simulink model "aaa"  (R2016b)
settings: Solver=ode4  StartTime=0.0  StopTime=inf  FixedStep=0.002  RelTol=1e-3  EnableMultiTasking=on
libraries: slrtlib x3
(part 2 of 5)

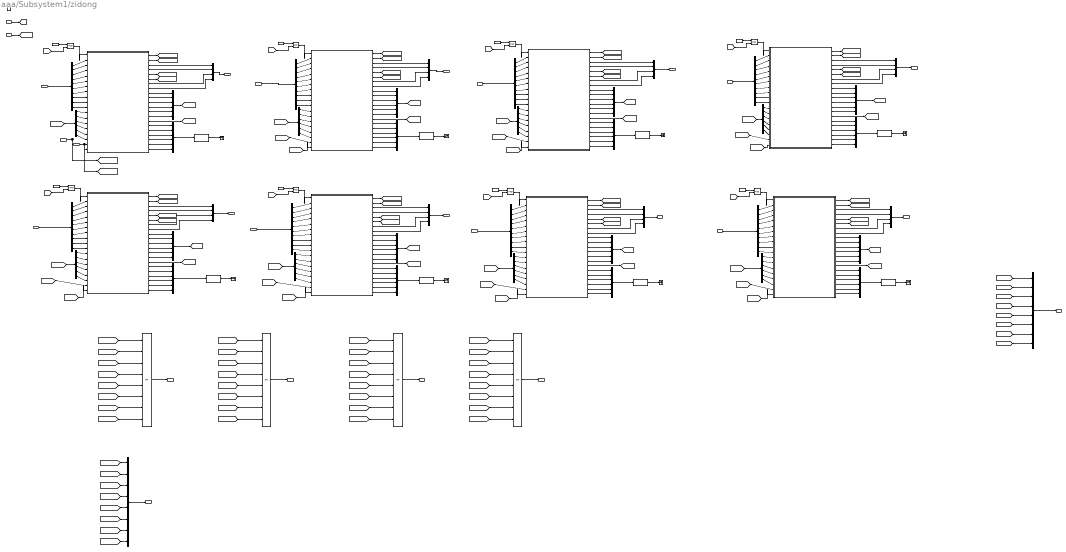
== system aaa/Subsystem1/zidong ==
  start : Inport
  In1 : Inport  Port=2
  In2 : Inport  Port=3
  In3 : Inport  Port=4
  In4 : Inport  Port=5
  In5 : Inport  Port=6
  In6 : Inport  Port=7
  In7 : Inport  Port=8
  In8 : Inport  Port=9
  "jiangeshijian " : Inport  Port=10
  shedingcishu : Inport  Port=11
  jieshu : Inport  Port=12
  Enable : EnablePort
  1# : Stateflow chart  TreatAsAtomicUnit=on
  1#1 : Stateflow chart  TreatAsAtomicUnit=on
  1#2 : Stateflow chart  TreatAsAtomicUnit=on
  1#3 : Stateflow chart  TreatAsAtomicUnit=on
  1#4 : Stateflow chart  TreatAsAtomicUnit=on
  1#5 : Stateflow chart  TreatAsAtomicUnit=on
  1#6 : Stateflow chart  TreatAsAtomicUnit=on
  1#7 : Stateflow chart  TreatAsAtomicUnit=on
  Data Type Conversion{1..8} (8 alike) : DataTypeConversion
  Demux{1..2,4,6,8,12,14,16} (8 alike) : Demux  Outputs=6
  Demux{3,5,7,9..11,13,15} (8 alike) : Demux  Outputs=10
  Logical Operator{,1..3} (4 alike) : Logic  Operator=OR  Inputs=8  AllPortsSameDT=off  OutDataTypeStr=boolean
  Logical Operator{4..11} (8 alike) : Logic  AllPortsSameDT=off  OutDataTypeStr=boolean
  Mux{,1..7} (8 alike) : Mux
  Mux{8..15,18..25} (16 alike) : Mux  Inputs=6
  Mux16 : Mux  Inputs=8
  Mux17 : Mux  Inputs=8
  Terminator{,1..7} (8 alike) : Terminator
  kaishi{1..8} (8 alike) : Constant  Value=0
      settings: OpenFcn=|
      | if get_param(gcb,'value')=='1',
      | set_param(gcb,'value','0');
      | else
      | set_param(gcb,'value','1');end
  songkaihuanxiang : Outport
  kaigaihuanxiang : Outport  Port=2
  yajinhuanxiang : Outport  Port=3
  guangaihuanxiang : Outport  Port=4
  Out1 : Outport  Port=5
  Out2 : Outport  Port=6
  Out3 : Outport  Port=7
  Out4 : Outport  Port=8
  Out5 : Outport  Port=9
  Out6 : Outport  Port=10
  Out7 : Outport  Port=11
  Out8 : Outport  Port=12
  "zidongshijian " : Outport  Port=13
  yikaicishu : Outport  Port=14
  wires:
  "jiangeshijian "/1 -> [jiangeshijian]
  Demux1/1 -> 1#/12(t1)
  Demux1/2 -> 1#/13(t3)
  Demux1/3 -> 1#/14(t5)
  Demux1/4 -> 1#/15(t7)
  Demux1/5 -> 1#/16(t9)
  [jiangeshijian] -> Demux1/1
  Demux9/1 -> 1#/2(kgdw1)
  Demux9/2 -> 1#/3(kgdw2)
  Demux9/3 -> 1#/4(ggdw1)
  Demux9/4 -> 1#/5(ggdw2)
  Demux9/5 -> 1#/6(kghc)
  Demux9/6 -> 1#/7(gghc)
  Demux9/7 -> 1#/8(sddw)
  Demux9/8 -> 1#/9(yjdw)
  Demux9/9 -> 1#/10(skdw)
  Demux9/10 -> 1#/11(jsdw)
  In1/1 -> Demux9/1  "kaigaidaowei1 kaigaidaowei2 guangaidaowei1 guangaidaowei2 kaigaihuanchong guangaihuanchong suodingdaowei jiesuodaowei yajindaowei songkaidaowei"
  start/1 -> [start]
  [start] -> Logical Operator4/2
  Demux2/1 -> 1#1/12(t1)
  Demux2/2 -> 1#1/13(t3)
  Demux2/3 -> 1#1/14(t5)
  Demux2/4 -> 1#1/15(t7)
  Demux2/5 -> 1#1/16(t9)
  [jiangeshijian] -> Demux2/1
  Demux3/1 -> 1#1/2(kgdw1)
  Demux3/2 -> 1#1/3(kgdw2)
  Demux3/3 -> 1#1/4(ggdw1)
  Demux3/4 -> 1#1/5(ggdw2)
  Demux3/5 -> 1#1/6(kghc)
  Demux3/6 -> 1#1/7(gghc)
  Demux3/7 -> 1#1/8(sddw)
  Demux3/8 -> 1#1/9(yjdw)
  Demux3/9 -> 1#1/10(skdw)
  Demux3/10 -> 1#1/11(jsdw)
  In2/1 -> Demux3/1  "kaigaidaowei1 kaigaidaowei2 guangaidaowei1 guangaidaowei2 kaigaihuanchong guangaihuanchong suodingdaowei jiesuodaowei yajindaowei songkaidaowei"
  [jiangeshijian] -> Demux4/1
  In3/1 -> Demux5/1  "kaigaidaowei1 kaigaidaowei2 guangaidaowei1 guangaidaowei2 kaigaihuanchong guangaihuanchong suodingdaowei jiesuodaowei yajindaowei songkaidaowei"
  [jiangeshijian] -> Demux6/1
  In4/1 -> Demux7/1  "kaigaidaowei1 kaigaidaowei2 guangaidaowei1 guangaidaowei2 kaigaihuanchong guangaihuanchong suodingdaowei jiesuodaowei yajindaowei songkaidaowei"
  [jiangeshijian] -> Demux8/1
  In5/1 -> Demux10/1  "kaigaidaowei1 kaigaidaowei2 guangaidaowei1 guangaidaowei2 kaigaihuanchong guangaihuanchong suodingdaowei jiesuodaowei yajindaowei songkaidaowei"
  [jiangeshijian] -> Demux12/1
  In6/1 -> Demux11/1  "kaigaidaowei1 kaigaidaowei2 guangaidaowei1 guangaidaowei2 kaigaihuanchong guangaihuanchong suodingdaowei jiesuodaowei yajindaowei songkaidaowei"
  [jiangeshijian] -> Demux14/1
  In7/1 -> Demux13/1  "kaigaidaowei1 kaigaidaowei2 guangaidaowei1 guangaidaowei2 kaigaihuanchong guangaihuanchong suodingdaowei jiesuodaowei yajindaowei songkaidaowei"
  [jiangeshijian] -> Demux16/1
  In8/1 -> Demux15/1  "kaigaidaowei1 kaigaidaowei2 guangaidaowei1 guangaidaowei2 kaigaihuanchong guangaihuanchong suodingdaowei jiesuodaowei yajindaowei songkaidaowei"
  Demux15/1 -> 1#7/2(kgdw1)
  Demux15/2 -> 1#7/3(kgdw2)
  Demux15/3 -> 1#7/4(ggdw1)
  Demux15/4 -> 1#7/5(ggdw2)
  Demux15/5 -> 1#7/6(kghc)
  Demux15/6 -> 1#7/7(gghc)
  Demux15/7 -> 1#7/8(sddw)
  Demux15/8 -> 1#7/9(yjdw)
  Demux15/9 -> 1#7/10(skdw)
  Demux15/10 -> 1#7/11(jsdw)
  Demux16/1 -> 1#7/12(t1)
  Demux16/2 -> 1#7/13(t3)
  Demux16/3 -> 1#7/14(t5)
  Demux16/4 -> 1#7/15(t7)
  Demux16/5 -> 1#7/16(t9)
  Demux13/1 -> 1#6/2(kgdw1)
  Demux13/2 -> 1#6/3(kgdw2)
  Demux13/3 -> 1#6/4(ggdw1)
  Demux13/4 -> 1#6/5(ggdw2)
  Demux13/5 -> 1#6/6(kghc)
  Demux13/6 -> 1#6/7(gghc)
  Demux13/7 -> 1#6/8(sddw)
  Demux13/8 -> 1#6/9(yjdw)
  Demux13/9 -> 1#6/10(skdw)
  Demux13/10 -> 1#6/11(jsdw)
  Demux14/1 -> 1#6/12(t1)
  Demux14/2 -> 1#6/13(t3)
  Demux14/3 -> 1#6/14(t5)
  Demux14/4 -> 1#6/15(t7)
  Demux14/5 -> 1#6/16(t9)
  Demux11/1 -> 1#5/2(kgdw1)
  Demux11/2 -> 1#5/3(kgdw2)
  Demux11/3 -> 1#5/4(ggdw1)
  Demux11/4 -> 1#5/5(ggdw2)
  Demux11/5 -> 1#5/6(kghc)
  Demux11/6 -> 1#5/7(gghc)
  Demux11/7 -> 1#5/8(sddw)
  Demux11/8 -> 1#5/9(yjdw)
  Demux11/9 -> 1#5/10(skdw)
  Demux11/10 -> 1#5/11(jsdw)
  Demux12/5 -> 1#5/16(t9)
  Demux12/4 -> 1#5/15(t7)
  Demux12/3 -> 1#5/14(t5)
  Demux12/1 -> 1#5/12(t1)
  Demux12/2 -> 1#5/13(t3)
  Demux8/1 -> 1#4/12(t1)
  Demux8/2 -> 1#4/13(t3)
  Demux8/3 -> 1#4/14(t5)
  Demux8/4 -> 1#4/15(t7)
  Demux8/5 -> 1#4/16(t9)
  Demux10/1 -> 1#4/2(kgdw1)
  Demux10/2 -> 1#4/3(kgdw2)
  Demux10/3 -> 1#4/4(ggdw1)
  Demux10/4 -> 1#4/5(ggdw2)
  Demux10/5 -> 1#4/6(kghc)
  Demux10/6 -> 1#4/7(gghc)
  Demux10/7 -> 1#4/8(sddw)
  Demux10/8 -> 1#4/9(yjdw)
  Demux10/9 -> 1#4/10(skdw)
  Demux10/10 -> 1#4/11(jsdw)
  Demux5/1 -> 1#2/2(kgdw1)
  Demux5/2 -> 1#2/3(kgdw2)
  Demux5/3 -> 1#2/4(ggdw1)
  Demux5/4 -> 1#2/5(ggdw2)
  Demux5/5 -> 1#2/6(kghc)
  Demux5/6 -> 1#2/7(gghc)
  Demux5/7 -> 1#2/8(sddw)
  Demux5/8 -> 1#2/9(yjdw)
  Demux5/9 -> 1#2/10(skdw)
  Demux5/10 -> 1#2/11(jsdw)
  Demux4/1 -> 1#2/12(t1)
  Demux4/2 -> 1#2/13(t3)
  Demux4/3 -> 1#2/14(t5)
  Demux4/4 -> 1#2/15(t7)
  Demux4/5 -> 1#2/16(t9)
  Demux7/1 -> 1#3/2(kgdw1)
  Demux7/2 -> 1#3/3(kgdw2)
  Demux7/3 -> 1#3/4(ggdw1)
  Demux7/4 -> 1#3/5(ggdw2)
  Demux7/5 -> 1#3/6(kghc)
  Demux7/6 -> 1#3/7(gghc)
  Demux7/7 -> 1#3/8(sddw)
  Demux7/8 -> 1#3/9(yjdw)
  Demux7/9 -> 1#3/10(skdw)
  Demux7/10 -> 1#3/11(jsdw)
  Demux6/1 -> 1#3/12(t1)
  Demux6/2 -> 1#3/13(t3)
  Demux6/3 -> 1#3/14(t5)
  Demux6/4 -> 1#3/15(t7)
  Demux6/5 -> 1#3/16(t9)
  1#/1(skhx) -> [songkaihuanxiang1]
  1#/2(kghx) -> [kaigaihuanxiang1]
  1#/5(yjhx) -> [yajinhuanxiang1]
  1#/6(gghx) -> [guangaihuanxiang1]
  1#1/1(skhx) -> [songkaihuanxiang2]
  1#1/2(kghx) -> [kaigaihuanxiang2]
  1#1/5(yjhx) -> [yajinhuanxiang2]
  1#1/6(gghx) -> [guangaihuanxiang2]
  1#2/1(skhx) -> [songkaihuanxiang3]
  1#2/2(kghx) -> [kaigaihuanxiang3]
  1#2/5(yjhx) -> [yajinhuanxiang3]
  1#2/6(gghx) -> [guangaihuanxiang3]
  1#4/2(kghx) -> [kaigaihuanxiang5]
  1#4/1(skhx) -> [songkaihuanxiang5]
  1#5/1(skhx) -> [songkaihuanxiang6]
  1#5/2(kghx) -> [kaigaihuanxiang6]
  1#7/1(skhx) -> [songkaihuanxiang8]
  1#7/2(kghx) -> [kaigaihuanxiang8]
  1#6/1(skhx) -> [songkaihuanxiang7]
  1#6/2(kghx) -> [kaigaihuanxiang7]
  1#6/5(yjhx) -> [yajinhuanxiang7]
  1#6/6(gghx) -> [guangaihuanxiang7]
  1#3/1(skhx) -> [songkaihuanxiang4]
  1#3/2(kghx) -> [kaigaihuanxiang4]
  [songkaihuanxiang1] -> Logical Operator/1
  [songkaihuanxiang2] -> Logical Operator/2
  [songkaihuanxiang3] -> Logical Operator/3
  [songkaihuanxiang4] -> Logical Operator/4
  [songkaihuanxiang5] -> Logical Operator/5
  [songkaihuanxiang8] -> Logical Operator/8
  [songkaihuanxiang7] -> Logical Operator/7
  [songkaihuanxiang6] -> Logical Operator/6
  Logical Operator/1 -> songkaihuanxiang/1
  [kaigaihuanxiang1] -> Logical Operator1/1
  [kaigaihuanxiang2] -> Logical Operator1/2
  [kaigaihuanxiang3] -> Logical Operator1/3
  [kaigaihuanxiang4] -> Logical Operator1/4
  [kaigaihuanxiang5] -> Logical Operator1/5
  [kaigaihuanxiang8] -> Logical Operator1/8
  [kaigaihuanxiang7] -> Logical Operator1/7
  [kaigaihuanxiang6] -> Logical Operator1/6
  Logical Operator1/1 -> kaigaihuanxiang/1
  [yajinhuanxiang1] -> Logical Operator2/1
  [yajinhuanxiang2] -> Logical Operator2/2
  [yajinhuanxiang3] -> Logical Operator2/3
  [yajinhuanxiang4] -> Logical Operator2/4
  [yajinhuanxiang5] -> Logical Operator2/5
  [yajinhuanxiang8] -> Logical Operator2/8
  [yajinhuanxiang7] -> Logical Operator2/7
  [yajinhuanxiang6] -> Logical Operator2/6
  Logical Operator2/1 -> yajinhuanxiang/1
  [guangaihuanxiang1] -> Logical Operator3/1
  [guangaihuanxiang2] -> Logical Operator3/2
  [guangaihuanxiang3] -> Logical Operator3/3
  [guangaihuanxiang4] -> Logical Operator3/4
  [guangaihuanxiang5] -> Logical Operator3/5
  [guangaihuanxiang8] -> Logical Operator3/8
  [guangaihuanxiang7] -> Logical Operator3/7
  [guangaihuanxiang6] -> Logical Operator3/6
  Logical Operator3/1 -> guangaihuanxiang/1
  1#/3(kgzhiling1) -> Mux/1
  1#/4(kgzhiling2) -> Mux/2
  1#/7(ggzhiling1) -> Mux/3
  1#/8(ggzhiling2) -> Mux/4
  1#1/7(ggzhiling1) -> Mux1/3
  Mux/1 -> Out1/1
  Mux1/1 -> Out2/1
  Mux2/1 -> Out3/1
  Mux4/1 -> Out5/1
  1#/9(skt) -> Mux8/1
  1#/10(kgt) -> Mux8/2
  1#/11(sdt) -> Mux8/3
  1#/12(jst) -> Mux8/4
  1#/13(ggt) -> Mux8/5
  1#/14(yjt) -> Mux8/6
  Mux8/1 -> [shijian1]
  Mux11/1 -> [shijian4]
  Mux21/1 -> [shijian5]
  [shijian1] -> Mux16/1
  [shijian2] -> Mux16/2
  [shijian3] -> Mux16/3
  [shijian4] -> Mux16/4
  [shijian5] -> Mux16/5
  [shijian6] -> Mux16/6
  [shijian7] -> Mux16/7
  Mux16/1 -> "zidongshijian "/1
  [shedingcishu] -> 1#5/18(shedingcishu)
  [shedingcishu] -> 1#6/18(shedingcishu)
  [shedingcishu] -> 1#7/18(shedingcishu)
  shedingcishu/1 -> 1#/18(shedingcishu), [shedingcishu]
  [shedingcishu] -> 1#4/18(shedingcishu)
  [shedingcishu] -> 1#1/18(shedingcishu)
  [shedingcishu] -> 1#2/18(shedingcishu)
  [shedingcishu] -> 1#3/18(shedingcishu)
  1#/15(yikaicishu) -> [yikaicishu1]
  1#1/15(yikaicishu) -> [yikaicishu2]
  1#2/15(yikaicishu) -> [yikaicishu3]
  [yikaicishu1] -> Mux17/1
  [yikaicishu4] -> Mux17/4
  [yikaicishu8] -> Mux17/8
  [yikaicishu7] -> Mux17/7
  [yikaicishu6] -> Mux17/6
  [yikaicishu5] -> Mux17/5
  [yikaicishu2] -> Mux17/2
  [yikaicishu3] -> Mux17/3
  Mux17/1 -> yikaicishu/1
  jieshu/1 -> 1#/19(jieshu), [jieshu]
  [jieshu] -> 1#1/19(jieshu)
  [jieshu] -> 1#2/19(jieshu)
  [jieshu] -> 1#3/19(jieshu)
  [jieshu] -> 1#7/19(jieshu)
  [jieshu] -> 1#4/19(jieshu)
  [jieshu] -> 1#5/19(jieshu)
  [jieshu] -> 1#6/19(jieshu)
  kaishi1/1 -> Logical Operator4/1
  Logical Operator4/1 -> 1#/1(start)
  [start] -> Logical Operator5/2
  kaishi2/1 -> Logical Operator5/1
  Logical Operator5/1 -> 1#1/1(start)
  [start] -> Logical Operator6/2
  kaishi3/1 -> Logical Operator6/1
  Logical Operator6/1 -> 1#2/1(start)
  [start] -> Logical Operator7/2
  kaishi4/1 -> Logical Operator7/1
  Logical Operator7/1 -> 1#3/1(start)
  [start] -> Logical Operator8/2
  kaishi5/1 -> Logical Operator8/1
  Logical Operator8/1 -> 1#4/1(start)
  [start] -> Logical Operator9/2
  kaishi6/1 -> Logical Operator9/1
  Logical Operator9/1 -> 1#5/1(start)
  [start] -> Logical Operator10/2
  kaishi7/1 -> Logical Operator10/1
  Logical Operator10/1 -> 1#6/1(start)
  [start] -> Logical Operator11/2
  kaishi8/1 -> Logical Operator11/1
  Logical Operator11/1 -> 1#7/1(start)
  Demux1/6 -> 1#/17(t11)
  Demux2/6 -> 1#1/17(t11)
  Demux4/6 -> 1#2/17(t11)
  Demux6/6 -> 1#3/17(t11)
  Demux8/6 -> 1#4/17(t11)
  Demux12/6 -> 1#5/17(t11)
  Demux14/6 -> 1#6/17(t11)
  Demux16/6 -> 1#7/17(t11)
  1#/16(skyichang) -> Mux18/1
  1#/17(kgyichang) -> Mux18/2
  1#/18(sdyichang) -> Mux18/3
  1#/19(jsyichang) -> Mux18/4
  1#/20(ggyichang) -> Mux18/5
  1#/21(yjyichang) -> Mux18/6
  Mux18/1 -> Data Type Conversion1/1
  Data Type Conversion1/1 -> Terminator/1
  1#1/3(kgzhiling1) -> Mux1/1
  1#1/4(kgzhiling2) -> Mux1/2
  1#1/8(ggzhiling2) -> Mux1/4
  1#1/9(skt) -> Mux9/1
  1#1/10(kgt) -> Mux9/2
  1#1/11(sdt) -> Mux9/3
  1#1/12(jst) -> Mux9/4
  1#1/13(ggt) -> Mux9/5
  1#1/14(yjt) -> Mux9/6
  Mux9/1 -> [shijian2]
  1#1/16(skyichang) -> Mux19/1
  1#1/17(kgyichang) -> Mux19/2
  1#1/18(sdyichang) -> Mux19/3
  1#1/19(jsyichang) -> Mux19/4
  1#1/20(ggyichang) -> Mux19/5
  1#1/21(yjyichang) -> Mux19/6
  Mux19/1 -> Data Type Conversion2/1
  Data Type Conversion2/1 -> Terminator1/1
  1#2/3(kgzhiling1) -> Mux2/1
  1#2/4(kgzhiling2) -> Mux2/2
  1#2/7(ggzhiling1) -> Mux2/3
  1#2/8(ggzhiling2) -> Mux2/4
  1#2/9(skt) -> Mux10/1
  1#2/10(kgt) -> Mux10/2
  1#2/11(sdt) -> Mux10/3
  1#2/12(jst) -> Mux10/4
  1#2/13(ggt) -> Mux10/5
  1#2/14(yjt) -> Mux10/6
  Mux10/1 -> [shijian3]
  1#2/16(skyichang) -> Mux20/1
  1#2/17(kgyichang) -> Mux20/2
  1#2/18(sdyichang) -> Mux20/3
  1#2/19(jsyichang) -> Mux20/4
  1#2/20(ggyichang) -> Mux20/5
  1#2/21(yjyichang) -> Mux20/6
  Mux20/1 -> Data Type Conversion3/1
  Data Type Conversion3/1 -> Terminator2/1
  1#3/5(yjhx) -> [yajinhuanxiang4]
  1#3/6(gghx) -> [guangaihuanxiang4]
  Mux3/1 -> Out4/1
  1#3/3(kgzhiling1) -> Mux3/1
  1#3/4(kgzhiling2) -> Mux3/2
  1#3/7(ggzhiling1) -> Mux3/3
  1#3/8(ggzhiling2) -> Mux3/4
  1#4/6(gghx) -> [guangaihuanxiang5]
  1#4/5(yjhx) -> [yajinhuanxiang5]
  1#4/3(kgzhiling1) -> Mux4/1
  1#4/4(kgzhiling2) -> Mux4/2
  1#4/7(ggzhiling1) -> Mux4/3
  1#4/8(ggzhiling2) -> Mux4/4
  1#4/9(skt) -> Mux21/1
  1#4/10(kgt) -> Mux21/2
  1#4/11(sdt) -> Mux21/3
  1#4/12(jst) -> Mux21/4
  1#4/13(ggt) -> Mux21/5
  1#4/14(yjt) -> Mux21/6
  1#4/15(yikaicishu) -> [yikaicishu5]
  1#4/17(kgyichang) -> Mux14/2
  1#4/18(sdyichang) -> Mux14/3
  1#4/19(jsyichang) -> Mux14/4
  1#4/20(ggyichang) -> Mux14/5
  1#4/21(yjyichang) -> Mux14/6
  1#4/16(skyichang) -> Mux14/1
  Mux14/1 -> Data Type Conversion4/1
  Data Type Conversion4/1 -> Terminator3/1
  1#5/15(yikaicishu) -> [yikaicishu6]
  1#5/5(yjhx) -> [yajinhuanxiang6]
  1#5/6(gghx) -> [guangaihuanxiang6]
  1#5/7(ggzhiling1) -> Mux5/3
  Mux5/1 -> Out6/1
  1#5/3(kgzhiling1) -> Mux5/1
  1#5/4(kgzhiling2) -> Mux5/2
  1#5/8(ggzhiling2) -> Mux5/4
  1#5/9(skt) -> Mux15/1
  1#5/10(kgt) -> Mux15/2
  1#5/11(sdt) -> Mux15/3
  1#5/12(jst) -> Mux15/4
  1#5/13(ggt) -> Mux15/5
  1#5/14(yjt) -> Mux15/6
  Mux15/1 -> [shijian6]
  1#5/16(skyichang) -> Mux22/1
  1#5/17(kgyichang) -> Mux22/2
  1#5/18(sdyichang) -> Mux22/3
  1#5/19(jsyichang) -> Mux22/4
  1#5/20(ggyichang) -> Mux22/5
  1#5/21(yjyichang) -> Mux22/6
  Mux22/1 -> Data Type Conversion5/1
  Data Type Conversion5/1 -> Terminator4/1
  1#6/7(ggzhiling1) -> Mux6/3
  Mux6/1 -> Out7/1
  1#6/3(kgzhiling1) -> Mux6/1
  1#6/4(kgzhiling2) -> Mux6/2
  1#6/8(ggzhiling2) -> Mux6/4
  1#6/9(skt) -> Mux12/1
  1#6/10(kgt) -> Mux12/2
  1#6/11(sdt) -> Mux12/3
  1#6/12(jst) -> Mux12/4
  1#6/13(ggt) -> Mux12/5
  1#6/14(yjt) -> Mux12/6
  Mux12/1 -> [shijian7]
  1#6/15(yikaicishu) -> [yikaicishu7]
  1#6/16(skyichang) -> Mux23/1
  1#6/17(kgyichang) -> Mux23/2
  1#6/18(sdyichang) -> Mux23/3
  1#6/19(jsyichang) -> Mux23/4
  1#6/20(ggyichang) -> Mux23/5
  1#6/21(yjyichang) -> Mux23/6
  Mux23/1 -> Data Type Conversion6/1
  Data Type Conversion6/1 -> Terminator5/1
  1#7/5(yjhx) -> [yajinhuanxiang8]
  1#7/6(gghx) -> [guangaihuanxiang8]
  1#7/7(ggzhiling1) -> Mux7/3
  Mux7/1 -> Out8/1
  1#7/3(kgzhiling1) -> Mux7/1
  1#7/4(kgzhiling2) -> Mux7/2
  1#7/8(ggzhiling2) -> Mux7/4
  1#7/9(skt) -> Mux13/1
  1#7/10(kgt) -> Mux13/2
  1#7/11(sdt) -> Mux13/3
  1#7/12(jst) -> Mux13/4
  1#7/13(ggt) -> Mux13/5
  1#7/14(yjt) -> Mux13/6
  Mux13/1 -> [shijian8]
  1#7/15(yikaicishu) -> [yikaicishu8]
  1#7/16(skyichang) -> Mux24/1
  1#7/17(kgyichang) -> Mux24/2
  1#7/18(sdyichang) -> Mux24/3
  1#7/19(jsyichang) -> Mux24/4
  1#7/20(ggyichang) -> Mux24/5
  1#7/21(yjyichang) -> Mux24/6
  Mux24/1 -> Data Type Conversion7/1
  Data Type Conversion7/1 -> Terminator6/1
  [shijian8] -> Mux16/8
  1#3/15(yikaicishu) -> [yikaicishu4]
  1#3/9(skt) -> Mux11/1
  1#3/10(kgt) -> Mux11/2
  1#3/11(sdt) -> Mux11/3
  1#3/12(jst) -> Mux11/4
  1#3/13(ggt) -> Mux11/5
  1#3/14(yjt) -> Mux11/6
  1#3/16(skyichang) -> Mux25/1
  1#3/17(kgyichang) -> Mux25/2
  1#3/18(sdyichang) -> Mux25/3
  1#3/19(jsyichang) -> Mux25/4
  1#3/20(ggyichang) -> Mux25/5
  1#3/21(yjyichang) -> Mux25/6
  Mux25/1 -> Data Type Conversion8/1
  Data Type Conversion8/1 -> Terminator7/1

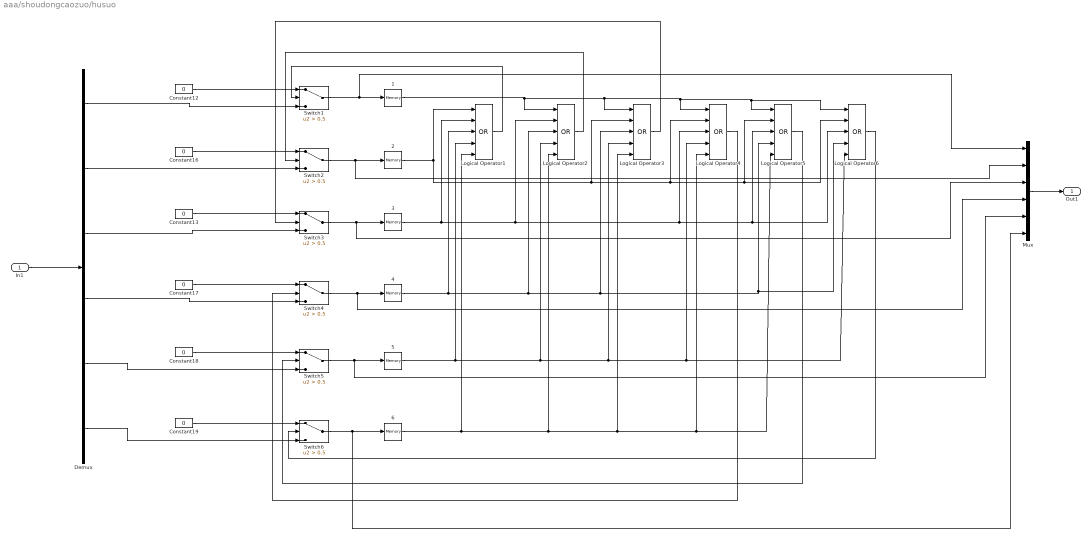
== system aaa/shoudongcaozuo/husuo ==
  In1 : Inport
  {1..6} (6 alike) : Memory
  Constant{12..13,16..19} (6 alike) : Constant  Value=0
  Demux : Demux  Outputs=6
  Logical Operator{1..6} (6 alike) : Logic  Operator=OR  Inputs=5  AllPortsSameDT=off  OutDataTypeStr=boolean
  Mux : Mux  Inputs=6
  Switch{1..6} (6 alike) : Switch  Criteria=u2 > Threshold  Threshold=0.5
  Out1 : Outport
  wires:
  In1/1 -> Demux/1
  Mux/1 -> Out1/1
  Constant16/1 -> Switch2/1
  Constant12/1 -> Switch1/1
  Constant17/1 -> Switch4/1
  Constant13/1 -> Switch3/1
  Constant19/1 -> Switch6/1
  Constant18/1 -> Switch5/1
  Switch1/1 -> Mux/1, 1/1
  Switch2/1 -> Mux/2, 2/1
  Switch3/1 -> Mux/3, 3/1
  Switch4/1 -> Mux/4, 4/1
  Switch5/1 -> Mux/5, 5/1
  Switch6/1 -> Mux/6, 6/1
  2/1 -> Logical Operator6/2, Logical Operator5/2, Logical Operator4/2, Logical Operator3/2, Logical Operator1/1
  3/1 -> Logical Operator6/3, Logical Operator5/3, Logical Operator4/3, Logical Operator2/2, Logical Operator1/2
  4/1 -> Logical Operator6/4, Logical Operator5/4, Logical Operator3/3, Logical Operator2/3, Logical Operator1/3
  5/1 -> Logical Operator6/5, Logical Operator4/4, Logical Operator3/4, Logical Operator2/4, Logical Operator1/4
  6/1 -> Logical Operator5/5, Logical Operator4/5, Logical Operator3/5, Logical Operator2/5, Logical Operator1/5
  1/1 -> Logical Operator6/1, Logical Operator5/1, Logical Operator4/1, Logical Operator3/1, Logical Operator2/1
  Logical Operator1/1 -> Switch1/2
  Logical Operator2/1 -> Switch2/2
  Logical Operator3/1 -> Switch3/2
  Logical Operator4/1 -> Switch4/2
  Logical Operator5/1 -> Switch5/2
  Logical Operator6/1 -> Switch6/2
  Demux/2 -> Switch2/3
  Demux/5 -> Switch5/3
  Demux/4 -> Switch4/3
  Demux/1 -> Switch1/3
  Demux/6 -> Switch6/3
  Demux/3 -> Switch3/3

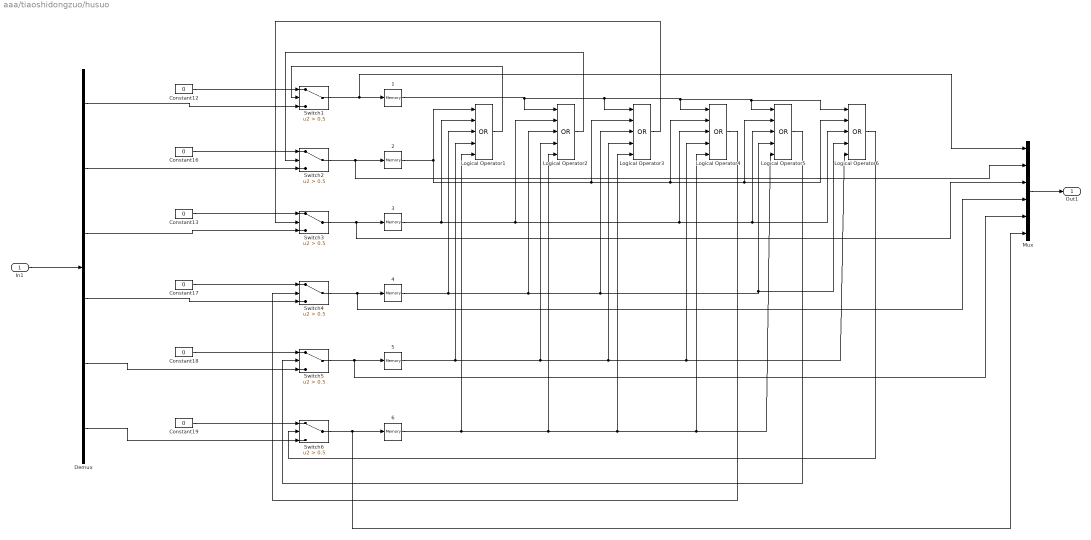
== system aaa/tiaoshidongzuo/husuo ==
  In1 : Inport
  {1..6} (6 alike) : Memory
  Constant{12..13,16..19} (6 alike) : Constant  Value=0
  Demux : Demux  Outputs=6
  Logical Operator{1..6} (6 alike) : Logic  Operator=OR  Inputs=5  AllPortsSameDT=off  OutDataTypeStr=boolean
  Mux : Mux  Inputs=6
  Switch{1..6} (6 alike) : Switch  Criteria=u2 > Threshold  Threshold=0.5
  Out1 : Outport
  wires:
  In1/1 -> Demux/1
  Mux/1 -> Out1/1
  Constant16/1 -> Switch2/1
  Constant12/1 -> Switch1/1
  Constant17/1 -> Switch4/1
  Constant13/1 -> Switch3/1
  Constant19/1 -> Switch6/1
  Constant18/1 -> Switch5/1
  Switch1/1 -> Mux/1, 1/1
  Switch2/1 -> Mux/2, 2/1
  Switch3/1 -> Mux/3, 3/1
  Switch4/1 -> Mux/4, 4/1
  Switch5/1 -> Mux/5, 5/1
  Switch6/1 -> Mux/6, 6/1
  2/1 -> Logical Operator6/2, Logical Operator5/2, Logical Operator4/2, Logical Operator3/2, Logical Operator1/1
  3/1 -> Logical Operator6/3, Logical Operator5/3, Logical Operator4/3, Logical Operator2/2, Logical Operator1/2
  4/1 -> Logical Operator6/4, Logical Operator5/4, Logical Operator3/3, Logical Operator2/3, Logical Operator1/3
  5/1 -> Logical Operator6/5, Logical Operator4/4, Logical Operator3/4, Logical Operator2/4, Logical Operator1/4
  6/1 -> Logical Operator5/5, Logical Operator4/5, Logical Operator3/5, Logical Operator2/5, Logical Operator1/5
  1/1 -> Logical Operator6/1, Logical Operator5/1, Logical Operator4/1, Logical Operator3/1, Logical Operator2/1
  Logical Operator1/1 -> Switch1/2
  Logical Operator2/1 -> Switch2/2
  Logical Operator3/1 -> Switch3/2
  Logical Operator4/1 -> Switch4/2
  Logical Operator5/1 -> Switch5/2
  Logical Operator6/1 -> Switch6/2
  Demux/2 -> Switch2/3
  Demux/5 -> Switch5/3
  Demux/4 -> Switch4/3
  Demux/1 -> Switch1/3
  Demux/6 -> Switch6/3
  Demux/3 -> Switch3/3

== stateflow chart aaa/Subsystem1/zidong/1# ==
  state zidong
    state chushihua
      entry:
      skhx=0;
      kghx=0;
      kgzhiling1=0;
      kgzhiling2=0;
      yjhx=0;
      gghx=0;
      ggzhiling1=0;
      ggzhiling2=0;
      skt=0;
      kgt=0;
      sdt=0;
      jst=0;
      ggt=0;
      yjt=0;
      skyichang=0;
      kgyichang=0;
      sdyichang=0;
      jsyichang=0;
      ggyichang=0;
      yjyichang=0;
    state on1
      entry:
      skhx=1;
    state songkaishijian
      entry:
      skt=skt+0.002;
    state start
      entry:
      yikaicishu = 0;
    state on10
      entry:
      skyichang=1;
    state songkaishijian1
      entry:
      skt=skt+0.002;
    state on8
      entry:
      skhx=0;
    state yanchishijian1
      entry:
      t=t+1;
    state tguiling
      entry: t=0;
    state on2
      entry:
      skhx=0;
      kghx=1;
      kgzhiling1=1;
      kgzhiling2=1;
    state kaigaishijian
      entry:
      kgt=kgt+0.002;
    state stop
      entry:
      skhx=0;
      kghx=0;
      kgzhiling1=0;
      kgzhiling2=0;
      yjhx=0;
      gghx=0;
      ggzhiling1=0;
      ggzhiling2=0;
      skt=0;
      kgt=0;
      sdt=0;
      jst=0;
      ggt=0;
      yjt=0;
    state songkaishijian2
      entry:
      kgt=kgt+0.002;
    state on9
      entry:
      kghx=0;
      kgzhiling1=0;
      kgzhiling2=0;
    state on11
      entry:
      kgyichang=1;
    state yanchishijian2
      entry:
      t2=t2+1;
    state t2guiling
      entry: t2=0;
    state on3
      entry:
      kghx=0;
      kgzhiling1=0;
      kgzhiling2=0;
      yjhx=1;
    state suodingshijian
      entry:
      sdt=sdt+0.002;
    state on7
      entry:
      yikaicishu = yikaicishu + 1;
    state songkaishijian3
      entry:
      sdt=sdt+0.002;
    state on13
      entry:
      yjhx=0;
    state on12
      entry:
      sdyichang=1;
    state yanchishijian3
      entry:
      t4=t4+1;
    state t4guiling
      entry: t4=0;
    state off
      entry:
      skhx=0;
      kghx=0;
      kgzhiling1=0;
      kgzhiling2=0;
      yjhx=0;
      gghx=0;
      ggzhiling1=0;
      ggzhiling2=0;
      skt=0;
      kgt=0;
      sdt=0;
      jst=0;
      ggt=0;
      yjt=0;
    state on4
      entry:
      yjhx=0;
      skhx=1;
    state jiesuoshijian
      entry:
      jst=jst+0.002;
    state songkaishijian4
      entry:
      jst=jst+0.002;
    state on15
      entry:
      skhx=0;
    state on14
      entry:
      jsyichang=1;
    state yanchishijian4
      entry:
      t6=t6+1;
    state t6guiling
      entry: t6=0;
    state on5
      entry:
      skhx=0;
      gghx=1;
      ggzhiling1=1;
      ggzhiling2=1;
    state guangaishijian
      entry:
      ggt=ggt+0.002;
    state songkaishijian5
      entry:
      ggt=ggt+0.002;
    state on17
      entry:
      gghx=0;
      ggzhiling1=0;
      ggzhiling2=0;
    state on16
      entry:
      ggyichang=1;
    state yanchishijian5
      entry:
      t8=t8+1;
    state t8guiling
      entry: t8=0;
    state yanchishijian6
      entry:
      t10=t10+1;
    state t10guiling
      entry: t10=0;
    state on6
      entry:
      gghx=0;
      ggzhiling1=0;
      ggzhiling2=0;
      yjhx=1;
    state yajinshijian
      entry:
      yjt=yjt+0.002;
    state songkaishijian6
      entry:
      yjt=yjt+0.002;
    state on19
      entry:
      yjhx=0;
    state on18
      entry:
      ggyichang=1;
    (default) -> start
    songkaishijian1 -> songkaishijian1 [order 1] : [jsdw==0||skdw==0]
    chushihua -> on1 : [start==1&&ggdw1==1&&ggdw2==1&&yjdw==1&&sddw==1]
    on1 -> (junction 48)
    (junction 48) -> songkaishijian [order 1] : [jsdw==0||skdw==0]
    start -> chushihua : [start==1]
    (junction 348) -> (junction 48) [order 1] : [skt<=2]
    (junction 48) -> tguiling [order 2] : [jsdw==1&&skdw==1]
    songkaishijian -> (junction 348)
    songkaishijian1 -> on8 [order 2] : [jsdw==1&&skdw==1]
    on10 -> songkaishijian1
    (junction 348) -> on10 [order 2] : [skt>2]
    (junction 54) -> yanchishijian1 [order 1] : [t<t1]
    yanchishijian1 -> (junction 54) : after(500,tick)
    tguiling -> (junction 54)
    (junction 54) -> on2 [order 2] : [t>=t1]
    (junction 190) -> chushihua [order 1] : [yikaicishu<shedingcishu&&jieshu==0]
    songkaishijian2 -> songkaishijian2 [order 1] : [kgdw1==0||kgdw2==0||jsdw==0||skdw==0]
    on2 -> (junction 65)
    (junction 65) -> kaigaishijian [order 1] : [kgdw1==0||kgdw2==0||jsdw==0||skdw==0]
    (junction 361) -> (junction 65) [order 2] : [kgt<=12]
    (junction 65) -> t2guiling [order 2] : [kgdw1==1&&kgdw2==1&&jsdw==1&&skdw==1]
    kaigaishijian -> (junction 361)
    (junction 76) -> yanchishijian2 [order 1] : [t2<t3]
    songkaishijian2 -> on9 [order 2] : [kgdw1==1&&kgdw2==1&&jsdw==1&&skdw==1]
    on11 -> songkaishijian2
    (junction 361) -> on11 [order 1] : [kgt>12]
    (junction 190) -> stop [order 2] : [yikaicishu>=shedingcishu||jieshu==1]
    on7 -> (junction 190)
    yanchishijian2 -> (junction 76) : after(500,tick)
    t2guiling -> (junction 76)
    (junction 76) -> on3 [order 2] : [t2>=t3]
    songkaishijian3 -> songkaishijian3 [order 1] : [kgdw1==0||kgdw2==0||sddw==0||yjdw==0]
    on3 -> (junction 96)
    (junction 96) -> suodingshijian [order 1] : [kgdw1==0||kgdw2==0||sddw==0||yjdw==0]
    (junction 386) -> (junction 96) [order 2] : [sdt<=2]
    (junction 96) -> t4guiling [order 2] : [kgdw1==1&&kgdw2==1&&sddw==1&&yjdw==1]
    off -> on7
    suodingshijian -> (junction 386)
    (junction 105) -> yanchishijian3 [order 1] : [t4<t5]
    songkaishijian3 -> on13 [order 2] : [kgdw1==1&&kgdw2==1&&jsdw==1&&skdw==1]
    on12 -> songkaishijian3
    (junction 386) -> on12 [order 1] : [sdt>2]
    yanchishijian3 -> (junction 105) : after(500,tick)
    t4guiling -> (junction 105)
    (junction 105) -> on4 [order 2] : [t4>=t5]
    songkaishijian4 -> songkaishijian4 [order 1] : [kgdw1==0||kgdw2==0||jsdw==0||skdw==0]
    on4 -> (junction 115)
    (junction 115) -> jiesuoshijian [order 1] : [kgdw1==0||kgdw2==0||jsdw==0||skdw==0]
    (junction 390) -> (junction 115) [order 2] : [jst<=2]
    (junction 115) -> t6guiling [order 2] : [kgdw1==1&&kgdw2==1&&jsdw==1&&skdw==1]
    jiesuoshijian -> (junction 390)
    (junction 125) -> yanchishijian4 [order 1] : [t6<t7]
    songkaishijian4 -> on15 [order 2] : [kgdw1==1&&kgdw2==1&&jsdw==1&&skdw==1]
    on14 -> songkaishijian4
    (junction 390) -> on14 [order 1] : [jst>2]
    yanchishijian4 -> (junction 125) : after(500,tick)
    t6guiling -> (junction 125)
    (junction 125) -> on5 [order 2] : [t6>=t7]
    (junction 339) -> off [order 2] : [t10>=t11]
    songkaishijian5 -> songkaishijian5 [order 2] : [ggdw1==0||ggdw2==0||jsdw==0||skdw==0]
    on5 -> (junction 142)
    (junction 142) -> guangaishijian [order 1] : [ggdw1==0||ggdw2==0||jsdw==0||skdw==0]
    (junction 403) -> (junction 142) [order 2] : [ggt<=12]
    (junction 142) -> t8guiling [order 2] : [ggdw1==1&&ggdw2==1&&jsdw==1&&skdw==1]
    guangaishijian -> (junction 403)
    (junction 154) -> yanchishijian5 [order 1] : [t8<t9]
    songkaishijian5 -> on17 [order 1] : [ggdw1==1&&ggdw2==1&&jsdw==1&&skdw==1]
    on16 -> songkaishijian5
    (junction 403) -> on16 [order 1] : [ggt>12]
    yanchishijian5 -> (junction 154) : after(500,tick)
    t8guiling -> (junction 154)
    (junction 154) -> on6 [order 2] : [t8>=t9]
    yanchishijian6 -> (junction 339) : after(500,tick)
    (junction 339) -> yanchishijian6 [order 1] : [t10<t11]
    t10guiling -> (junction 339)
    (junction 162) -> t10guiling [order 2] : [sddw==1&&yjdw==1&&ggdw1==1&&ggdw2==1]
    on6 -> (junction 162)
    (junction 162) -> yajinshijian [order 1] : [sddw==0||yjdw==0]
    songkaishijian6 -> songkaishijian6 [order 2] : [sddw==0||yjdw==0]
    (junction 410) -> (junction 162) [order 2] : [yjt<=2]
    yajinshijian -> (junction 410)
    songkaishijian6 -> on19 [order 1] : [sddw==1&&yjdw==1&&ggdw1==1&&ggdw2==1]
    on18 -> songkaishijian6
    (junction 410) -> on18 [order 1] : [yjt>2]
  (default) -> zidong
  data: start input; kgdw1 input; kgdw2 input; skhx output; kghx output; kgzhiling1 output; kgzhiling2 output; yjhx output; gghx output; ggzhiling1 output; ggzhiling2 output; skt output; kgt output; sdt output; jst output; ggt output; yjt output; ggdw1 input; ggdw2 input; kghc input; gghc input; sddw input; yjdw input; skdw input; jsdw input; t1 input; t3 input; t5 input; t7 input; t9 input; t11 input; t local; t2 local; t4 local; t6 local; t8 local; shedingcishu input; yikaicishu output; skyichang output; kgyichang output; sdyichang output; jsyichang output; jieshu input; t10 local; ggyichang output; yjyichang output

== stateflow chart aaa/Subsystem1/zidong/1#1 ==
  state zidong
    state chushihua
      entry:
      skhx=0;
      kghx=0;
      kgzhiling1=0;
      kgzhiling2=0;
      yjhx=0;
      gghx=0;
      ggzhiling1=0;
      ggzhiling2=0;
      skt=0;
      kgt=0;
      sdt=0;
      jst=0;
      ggt=0;
      yjt=0;
      skyichang=0;
      kgyichang=0;
      sdyichang=0;
      jsyichang=0;
      ggyichang=0;
      yjyichang=0;
    state on1
      entry:
      skhx=1;
    state songkaishijian
      entry:
      skt=skt+0.002;
    state start
      entry:
      yikaicishu = 0;
    state on10
      entry:
      skyichang=1;
    state songkaishijian1
      entry:
      skt=skt+0.002;
    state on8
      entry:
      skhx=0;
    state yanchishijian1
      entry:
      t=t+1;
    state tguiling
      entry: t=0;
    state on2
      entry:
      skhx=0;
      kghx=1;
      kgzhiling1=1;
      kgzhiling2=1;
    state kaigaishijian
      entry:
      kgt=kgt+0.002;
    state stop
      entry:
      skhx=0;
      kghx=0;
      kgzhiling1=0;
      kgzhiling2=0;
      yjhx=0;
      gghx=0;
      ggzhiling1=0;
      ggzhiling2=0;
      skt=0;
      kgt=0;
      sdt=0;
      jst=0;
      ggt=0;
      yjt=0;
    state songkaishijian2
      entry:
      kgt=kgt+0.002;
    state on9
      entry:
      kghx=0;
      kgzhiling1=0;
      kgzhiling2=0;
    state on11
      entry:
      kgyichang=1;
    state yanchishijian2
      entry:
      t2=t2+1;
    state t2guiling
      entry: t2=0;
    state on3
      entry:
      kghx=0;
      kgzhiling1=0;
      kgzhiling2=0;
      yjhx=1;
    state suodingshijian
      entry:
      sdt=sdt+0.002;
    state on7
      entry:
      yikaicishu = yikaicishu + 1;
    state songkaishijian3
      entry:
      sdt=sdt+0.002;
    state on13
      entry:
      yjhx=0;
    state on12
      entry:
      sdyichang=1;
    state yanchishijian3
      entry:
      t4=t4+1;
    state t4guiling
      entry: t4=0;
    state off
      entry:
      skhx=0;
      kghx=0;
      kgzhiling1=0;
      kgzhiling2=0;
      yjhx=0;
      gghx=0;
      ggzhiling1=0;
      ggzhiling2=0;
      skt=0;
      kgt=0;
      sdt=0;
      jst=0;
      ggt=0;
      yjt=0;
    state on4
      entry:
      yjhx=0;
      skhx=1;
    state jiesuoshijian
      entry:
      jst=jst+0.002;
    state songkaishijian4
      entry:
      jst=jst+0.002;
    state on15
      entry:
      skhx=0;
    state on14
      entry:
      jsyichang=1;
    state yanchishijian4
      entry:
      t6=t6+1;
    state t6guiling
      entry: t6=0;
    state on5
      entry:
      skhx=0;
      gghx=1;
      ggzhiling1=1;
      ggzhiling2=1;
    state guangaishijian
      entry:
      ggt=ggt+0.002;
    state songkaishijian5
      entry:
      ggt=ggt+0.002;
    state on17
      entry:
      gghx=0;
      ggzhiling1=0;
      ggzhiling2=0;
    state on16
      entry:
      ggyichang=1;
    state yanchishijian5
      entry:
      t8=t8+1;
    state t8guiling
      entry: t8=0;
    state yanchishijian6
      entry:
      t10=t10+1;
    state t10guiling
      entry: t10=0;
    state on6
      entry:
      gghx=0;
      ggzhiling1=0;
      ggzhiling2=0;
      yjhx=1;
    state yajinshijian
      entry:
      yjt=yjt+0.002;
    state songkaishijian6
      entry:
      yjt=yjt+0.002;
    state on19
      entry:
      yjhx=0;
    state on18
      entry:
      ggyichang=1;
    (default) -> start
    songkaishijian1 -> songkaishijian1 [order 1] : [jsdw==0||skdw==0]
    chushihua -> on1 : [start==1&&ggdw1==1&&ggdw2==1&&yjdw==1&&sddw==1]
    on1 -> (junction 48)
    (junction 48) -> songkaishijian [order 1] : [jsdw==0||skdw==0]
    start -> chushihua : [start==1]
    (junction 348) -> (junction 48) [order 1] : [skt<=2]
    (junction 48) -> tguiling [order 2] : [jsdw==1&&skdw==1]
    songkaishijian -> (junction 348)
    songkaishijian1 -> on8 [order 2] : [jsdw==1&&skdw==1]
    on10 -> songkaishijian1
    (junction 348) -> on10 [order 2] : [skt>2]
    (junction 54) -> yanchishijian1 [order 1] : [t<t1]
    yanchishijian1 -> (junction 54) : after(500,tick)
    tguiling -> (junction 54)
    (junction 54) -> on2 [order 2] : [t>=t1]
    (junction 190) -> chushihua [order 1] : [yikaicishu<shedingcishu&&jieshu==0]
    songkaishijian2 -> songkaishijian2 [order 1] : [kgdw1==0||kgdw2==0||jsdw==0||skdw==0]
    on2 -> (junction 65)
    (junction 65) -> kaigaishijian [order 1] : [kgdw1==0||kgdw2==0||jsdw==0||skdw==0]
    (junction 361) -> (junction 65) [order 2] : [kgt<=12]
    (junction 65) -> t2guiling [order 2] : [kgdw1==1&&kgdw2==1&&jsdw==1&&skdw==1]
    kaigaishijian -> (junction 361)
    (junction 76) -> yanchishijian2 [order 1] : [t2<t3]
    songkaishijian2 -> on9 [order 2] : [kgdw1==1&&kgdw2==1&&jsdw==1&&skdw==1]
    on11 -> songkaishijian2
    (junction 361) -> on11 [order 1] : [kgt>12]
    (junction 190) -> stop [order 2] : [yikaicishu>=shedingcishu||jieshu==1]
    on7 -> (junction 190)
    yanchishijian2 -> (junction 76) : after(500,tick)
    t2guiling -> (junction 76)
    (junction 76) -> on3 [order 2] : [t2>=t3]
    songkaishijian3 -> songkaishijian3 [order 1] : [kgdw1==0||kgdw2==0||sddw==0||yjdw==0]
    on3 -> (junction 96)
    (junction 96) -> suodingshijian [order 1] : [kgdw1==0||kgdw2==0||sddw==0||yjdw==0]
    (junction 386) -> (junction 96) [order 2] : [sdt<=2]
    (junction 96) -> t4guiling [order 2] : [kgdw1==1&&kgdw2==1&&sddw==1&&yjdw==1]
    off -> on7
    suodingshijian -> (junction 386)
    (junction 105) -> yanchishijian3 [order 1] : [t4<t5]
    songkaishijian3 -> on13 [order 2] : [kgdw1==1&&kgdw2==1&&jsdw==1&&skdw==1]
    on12 -> songkaishijian3
    (junction 386) -> on12 [order 1] : [sdt>2]
    yanchishijian3 -> (junction 105) : after(500,tick)
    t4guiling -> (junction 105)
    (junction 105) -> on4 [order 2] : [t4>=t5]
    songkaishijian4 -> songkaishijian4 [order 1] : [kgdw1==0||kgdw2==0||jsdw==0||skdw==0]
    on4 -> (junction 115)
    (junction 115) -> jiesuoshijian [order 1] : [kgdw1==0||kgdw2==0||jsdw==0||skdw==0]
    (junction 390) -> (junction 115) [order 2] : [jst<=2]
    (junction 115) -> t6guiling [order 2] : [kgdw1==1&&kgdw2==1&&jsdw==1&&skdw==1]
    jiesuoshijian -> (junction 390)
    (junction 125) -> yanchishijian4 [order 1] : [t6<t7]
    songkaishijian4 -> on15 [order 2] : [kgdw1==1&&kgdw2==1&&jsdw==1&&skdw==1]
    on14 -> songkaishijian4
    (junction 390) -> on14 [order 1] : [jst>2]
    yanchishijian4 -> (junction 125) : after(500,tick)
    t6guiling -> (junction 125)
    (junction 125) -> on5 [order 2] : [t6>=t7]
    (junction 339) -> off [order 2] : [t10>=t11]
    songkaishijian5 -> songkaishijian5 [order 2] : [ggdw1==0||ggdw2==0||jsdw==0||skdw==0]
    on5 -> (junction 142)
    (junction 142) -> guangaishijian [order 1] : [ggdw1==0||ggdw2==0||jsdw==0||skdw==0]
    (junction 403) -> (junction 142) [order 2] : [ggt<=12]
    (junction 142) -> t8guiling [order 2] : [ggdw1==1&&ggdw2==1&&jsdw==1&&skdw==1]
    guangaishijian -> (junction 403)
    (junction 154) -> yanchishijian5 [order 1] : [t8<t9]
    songkaishijian5 -> on17 [order 1] : [ggdw1==1&&ggdw2==1&&jsdw==1&&skdw==1]
    on16 -> songkaishijian5
    (junction 403) -> on16 [order 1] : [ggt>12]
    yanchishijian5 -> (junction 154) : after(500,tick)
    t8guiling -> (junction 154)
    (junction 154) -> on6 [order 2] : [t8>=t9]
    yanchishijian6 -> (junction 339) : after(500,tick)
    (junction 339) -> yanchishijian6 [order 1] : [t10<t11]
    t10guiling -> (junction 339)
    (junction 162) -> t10guiling [order 2] : [sddw==1&&yjdw==1&&ggdw1==1&&ggdw2==1]
    on6 -> (junction 162)
    (junction 162) -> yajinshijian [order 1] : [sddw==0||yjdw==0]
    songkaishijian6 -> songkaishijian6 [order 2] : [sddw==0||yjdw==0]
    (junction 410) -> (junction 162) [order 2] : [yjt<=2]
    yajinshijian -> (junction 410)
    songkaishijian6 -> on19 [order 1] : [sddw==1&&yjdw==1&&ggdw1==1&&ggdw2==1]
    on18 -> songkaishijian6
    (junction 410) -> on18 [order 1] : [yjt>2]
  (default) -> zidong
  data: start input; kgdw1 input; kgdw2 input; skhx output; kghx output; kgzhiling1 output; kgzhiling2 output; yjhx output; gghx output; ggzhiling1 output; ggzhiling2 output; skt output; kgt output; sdt output; jst output; ggt output; yjt output; ggdw1 input; ggdw2 input; kghc input; gghc input; sddw input; yjdw input; skdw input; jsdw input; t1 input; t3 input; t5 input; t7 input; t9 input; t11 input; t local; t2 local; t4 local; t6 local; t8 local; shedingcishu input; yikaicishu output; skyichang output; kgyichang output; sdyichang output; jsyichang output; jieshu input; t10 local; ggyichang output; yjyichang output

== stateflow chart aaa/Subsystem1/zidong/1#2 ==
  state zidong
    state chushihua
      entry:
      skhx=0;
      kghx=0;
      kgzhiling1=0;
      kgzhiling2=0;
      yjhx=0;
      gghx=0;
      ggzhiling1=0;
      ggzhiling2=0;
      skt=0;
      kgt=0;
      sdt=0;
      jst=0;
      ggt=0;
      yjt=0;
      skyichang=0;
      kgyichang=0;
      sdyichang=0;
      jsyichang=0;
      ggyichang=0;
      yjyichang=0;
    state on1
      entry:
      skhx=1;
    state songkaishijian
      entry:
      skt=skt+0.002;
    state start
      entry:
      yikaicishu = 0;
    state on10
      entry:
      skyichang=1;
    state songkaishijian1
      entry:
      skt=skt+0.002;
    state on8
      entry:
      skhx=0;
    state yanchishijian1
      entry:
      t=t+1;
    state tguiling
      entry: t=0;
    state on2
      entry:
      skhx=0;
      kghx=1;
      kgzhiling1=1;
      kgzhiling2=1;
    state kaigaishijian
      entry:
      kgt=kgt+0.002;
    state stop
      entry:
      skhx=0;
      kghx=0;
      kgzhiling1=0;
      kgzhiling2=0;
      yjhx=0;
      gghx=0;
      ggzhiling1=0;
      ggzhiling2=0;
      skt=0;
      kgt=0;
      sdt=0;
      jst=0;
      ggt=0;
      yjt=0;
    state songkaishijian2
      entry:
      kgt=kgt+0.002;
    state on9
      entry:
      kghx=0;
      kgzhiling1=0;
      kgzhiling2=0;
    state on11
      entry:
      kgyichang=1;
    state yanchishijian2
      entry:
      t2=t2+1;
    state t2guiling
      entry: t2=0;
    state on3
      entry:
      kghx=0;
      kgzhiling1=0;
      kgzhiling2=0;
      yjhx=1;
    state suodingshijian
      entry:
      sdt=sdt+0.002;
    state on7
      entry:
      yikaicishu = yikaicishu + 1;
    state songkaishijian3
      entry:
      sdt=sdt+0.002;
    state on13
      entry:
      yjhx=0;
    state on12
      entry:
      sdyichang=1;
    state yanchishijian3
      entry:
      t4=t4+1;
    state t4guiling
      entry: t4=0;
    state off
      entry:
      skhx=0;
      kghx=0;
      kgzhiling1=0;
      kgzhiling2=0;
      yjhx=0;
      gghx=0;
      ggzhiling1=0;
      ggzhiling2=0;
      skt=0;
      kgt=0;
      sdt=0;
      jst=0;
      ggt=0;
      yjt=0;
    state on4
      entry:
      yjhx=0;
      skhx=1;
    state jiesuoshijian
      entry:
      jst=jst+0.002;
    state songkaishijian4
      entry:
      jst=jst+0.002;
    state on15
      entry:
      skhx=0;
    state on14
      entry:
      jsyichang=1;
    state yanchishijian4
      entry:
      t6=t6+1;
    state t6guiling
      entry: t6=0;
    state on5
      entry:
      skhx=0;
      gghx=1;
      ggzhiling1=1;
      ggzhiling2=1;
    state guangaishijian
      entry:
      ggt=ggt+0.002;
    state songkaishijian5
      entry:
      ggt=ggt+0.002;
    state on17
      entry:
      gghx=0;
      ggzhiling1=0;
      ggzhiling2=0;
    state on16
      entry:
      ggyichang=1;
    state yanchishijian5
      entry:
      t8=t8+1;
    state t8guiling
      entry: t8=0;
    state yanchishijian6
      entry:
      t10=t10+1;
    state t10guiling
      entry: t10=0;
    state on6
      entry:
      gghx=0;
      ggzhiling1=0;
      ggzhiling2=0;
      yjhx=1;
    state yajinshijian
      entry:
      yjt=yjt+0.002;
    state songkaishijian6
      entry:
      yjt=yjt+0.002;
    state on19
      entry:
      yjhx=0;
    state on18
      entry:
      ggyichang=1;
    (default) -> start
    songkaishijian1 -> songkaishijian1 [order 1] : [jsdw==0||skdw==0]
    chushihua -> on1 : [start==1&&ggdw1==1&&ggdw2==1&&yjdw==1&&sddw==1]
    on1 -> (junction 48)
    (junction 48) -> songkaishijian [order 1] : [jsdw==0||skdw==0]
    start -> chushihua : [start==1]
    (junction 348) -> (junction 48) [order 1] : [skt<=2]
    (junction 48) -> tguiling [order 2] : [jsdw==1&&skdw==1]
    songkaishijian -> (junction 348)
    songkaishijian1 -> on8 [order 2] : [jsdw==1&&skdw==1]
    on10 -> songkaishijian1
    (junction 348) -> on10 [order 2] : [skt>2]
    (junction 54) -> yanchishijian1 [order 1] : [t<t1]
    yanchishijian1 -> (junction 54) : after(500,tick)
    tguiling -> (junction 54)
    (junction 54) -> on2 [order 2] : [t>=t1]
    (junction 190) -> chushihua [order 1] : [yikaicishu<shedingcishu&&jieshu==0]
    songkaishijian2 -> songkaishijian2 [order 1] : [kgdw1==0||kgdw2==0||jsdw==0||skdw==0]
    on2 -> (junction 65)
    (junction 65) -> kaigaishijian [order 1] : [kgdw1==0||kgdw2==0||jsdw==0||skdw==0]
    (junction 361) -> (junction 65) [order 2] : [kgt<=12]
    (junction 65) -> t2guiling [order 2] : [kgdw1==1&&kgdw2==1&&jsdw==1&&skdw==1]
    kaigaishijian -> (junction 361)
    (junction 76) -> yanchishijian2 [order 1] : [t2<t3]
    songkaishijian2 -> on9 [order 2] : [kgdw1==1&&kgdw2==1&&jsdw==1&&skdw==1]
    on11 -> songkaishijian2
    (junction 361) -> on11 [order 1] : [kgt>12]
    (junction 190) -> stop [order 2] : [yikaicishu>=shedingcishu||jieshu==1]
    on7 -> (junction 190)
    yanchishijian2 -> (junction 76) : after(500,tick)
    t2guiling -> (junction 76)
    (junction 76) -> on3 [order 2] : [t2>=t3]
    songkaishijian3 -> songkaishijian3 [order 1] : [kgdw1==0||kgdw2==0||sddw==0||yjdw==0]
    on3 -> (junction 96)
    (junction 96) -> suodingshijian [order 1] : [kgdw1==0||kgdw2==0||sddw==0||yjdw==0]
    (junction 386) -> (junction 96) [order 2] : [sdt<=2]
    (junction 96) -> t4guiling [order 2] : [kgdw1==1&&kgdw2==1&&sddw==1&&yjdw==1]
    off -> on7
    suodingshijian -> (junction 386)
    (junction 105) -> yanchishijian3 [order 1] : [t4<t5]
    songkaishijian3 -> on13 [order 2] : [kgdw1==1&&kgdw2==1&&jsdw==1&&skdw==1]
    on12 -> songkaishijian3
    (junction 386) -> on12 [order 1] : [sdt>2]
    yanchishijian3 -> (junction 105) : after(500,tick)
    t4guiling -> (junction 105)
    (junction 105) -> on4 [order 2] : [t4>=t5]
    songkaishijian4 -> songkaishijian4 [order 1] : [kgdw1==0||kgdw2==0||jsdw==0||skdw==0]
    on4 -> (junction 115)
    (junction 115) -> jiesuoshijian [order 1] : [kgdw1==0||kgdw2==0||jsdw==0||skdw==0]
    (junction 390) -> (junction 115) [order 2] : [jst<=2]
    (junction 115) -> t6guiling [order 2] : [kgdw1==1&&kgdw2==1&&jsdw==1&&skdw==1]
    jiesuoshijian -> (junction 390)
    (junction 125) -> yanchishijian4 [order 1] : [t6<t7]
    songkaishijian4 -> on15 [order 2] : [kgdw1==1&&kgdw2==1&&jsdw==1&&skdw==1]
    on14 -> songkaishijian4
    (junction 390) -> on14 [order 1] : [jst>2]
    yanchishijian4 -> (junction 125) : after(500,tick)
    t6guiling -> (junction 125)
    (junction 125) -> on5 [order 2] : [t6>=t7]
    (junction 339) -> off [order 2] : [t10>=t11]
    songkaishijian5 -> songkaishijian5 [order 2] : [ggdw1==0||ggdw2==0||jsdw==0||skdw==0]
    on5 -> (junction 142)
    (junction 142) -> guangaishijian [order 1] : [ggdw1==0||ggdw2==0||jsdw==0||skdw==0]
    (junction 403) -> (junction 142) [order 2] : [ggt<=12]
    (junction 142) -> t8guiling [order 2] : [ggdw1==1&&ggdw2==1&&jsdw==1&&skdw==1]
    guangaishijian -> (junction 403)
    (junction 154) -> yanchishijian5 [order 1] : [t8<t9]
    songkaishijian5 -> on17 [order 1] : [ggdw1==1&&ggdw2==1&&jsdw==1&&skdw==1]
    on16 -> songkaishijian5
    (junction 403) -> on16 [order 1] : [ggt>12]
    yanchishijian5 -> (junction 154) : after(500,tick)
    t8guiling -> (junction 154)
    (junction 154) -> on6 [order 2] : [t8>=t9]
    yanchishijian6 -> (junction 339) : after(500,tick)
    (junction 339) -> yanchishijian6 [order 1] : [t10<t11]
    t10guiling -> (junction 339)
    (junction 162) -> t10guiling [order 2] : [sddw==1&&yjdw==1&&ggdw1==1&&ggdw2==1]
    on6 -> (junction 162)
    (junction 162) -> yajinshijian [order 1] : [sddw==0||yjdw==0]
    songkaishijian6 -> songkaishijian6 [order 2] : [sddw==0||yjdw==0]
    (junction 410) -> (junction 162) [order 2] : [yjt<=2]
    yajinshijian -> (junction 410)
    songkaishijian6 -> on19 [order 1] : [sddw==1&&yjdw==1&&ggdw1==1&&ggdw2==1]
    on18 -> songkaishijian6
    (junction 410) -> on18 [order 1] : [yjt>2]
  (default) -> zidong
  data: start input; kgdw1 input; kgdw2 input; skhx output; kghx output; kgzhiling1 output; kgzhiling2 output; yjhx output; gghx output; ggzhiling1 output; ggzhiling2 output; skt output; kgt output; sdt output; jst output; ggt output; yjt output; ggdw1 input; ggdw2 input; kghc input; gghc input; sddw input; yjdw input; skdw input; jsdw input; t1 input; t3 input; t5 input; t7 input; t9 input; t11 input; t local; t2 local; t4 local; t6 local; t8 local; shedingcishu input; yikaicishu output; skyichang output; kgyichang output; sdyichang output; jsyichang output; jieshu input; t10 local; ggyichang output; yjyichang output
